simulink model "Example3_Calibrating_The_AR_Drone_Model"  (R2016a)
settings: configuration reference "AR_Drone_ConfigSet" (kept outside this file)
libraries: simulink x1, AR_Drone_2_Library x1, ARdrone_video_lib x1
settings Model: SimulationMode=external  Creator=sannem  LastModifiedBy=sannem
settings ConfigSetRef: SourceLocation=Base Workspace

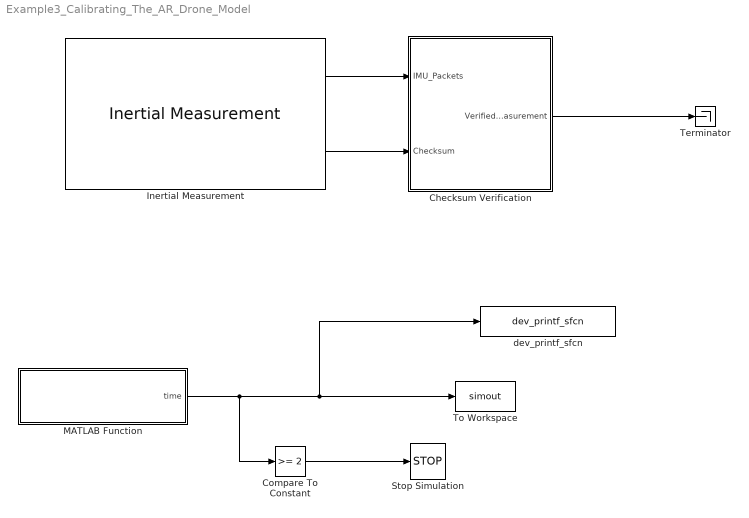
== system Example3_Calibrating_The_AR_Drone_Model ==
  Checksum Verification : Subsystem
  Compare To Constant : simulink/Logic and Bit Operations/Compare To Constant  relop=>=  const=2  OutDataTypeStr=boolean
  Inertial Measurement : AR_Drone_2_Library/Inertial Measurement  Ts=1/400
  MATLAB Function : MATLAB Function  TreatAsAtomicUnit=on
  Stop Simulation : Stop
  Terminator : Terminator
  To Workspace : ToWorkspace  VariableName=simout  SaveFormat=Structure With Time  SampleTime=-1
  dev_printf_sfcn : ARdrone_video_lib/dev_printf_sfcn  SFunctionSpec=ARpintf_Update(double u1)  SampleTime=-1  ShowSpec=on
  wires:
  Inertial Measurement/1 -> Checksum Verification/1(IMU_Packets)
  Inertial Measurement/2 -> Checksum Verification/2(Checksum)
  Checksum Verification/1(Verified_Raw_Measurement) -> Terminator/1
  MATLAB Function/1(time) -> Compare To Constant/1, To Workspace/1, dev_printf_sfcn/1
  Compare To Constant/1 -> Stop Simulation/1

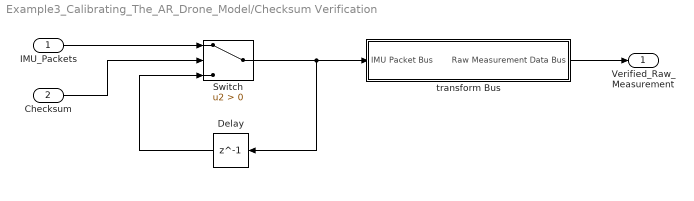
== system Example3_Calibrating_The_AR_Drone_Model/Checksum Verification ==
  IMU_Packets : Inport
  Checksum : Inport  Port=2
  Delay : Delay  DelayLength=1
  Switch : Switch  Criteria=u2 > Threshold
  transform Bus : Subsystem
  Verified_Raw_Measurement : Outport
  wires:
  IMU_Packets/1 -> Switch/1
  transform Bus/1(Raw Measurement Data Bus) -> Verified_Raw_Measurement/1
  Checksum/1 -> Switch/2
  Delay/1 -> Switch/3
  Switch/1 -> Delay/1, transform Bus/1(IMU Packet Bus)

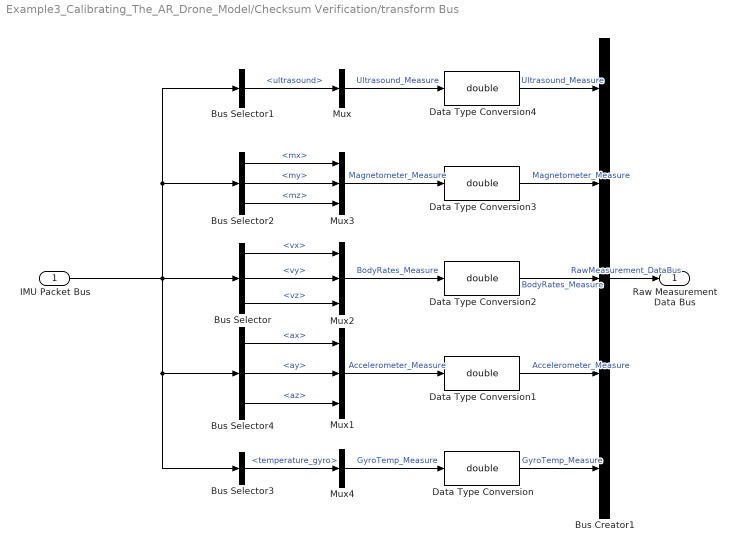
== system Example3_Calibrating_The_AR_Drone_Model/Checksum Verification/transform Bus ==
  IMU Packet Bus : Inport  OutDataTypeStr=Bus: IMU_Packets
  Bus Creator1 : BusCreator  Inputs='Ultrasound_Measure','Magnetometer_Measure','BodyRates_Measure','Accelerometer_Measure','GyroTemp_Measure'
  Bus Selector : BusSelector  OutputSignals=vx,vy,vz
  Bus Selector1 : BusSelector  OutputSignals=ultrasound
  Bus Selector2 : BusSelector  OutputSignals=mx,my,mz
  Bus Selector3 : BusSelector  OutputSignals=temperature_gyro
  Bus Selector4 : BusSelector  OutputSignals=ax,ay,az
  Data Type Conversion{,1..4} (5 alike) : DataTypeConversion  OutDataTypeStr=double
  Mux : Mux  Inputs=1
  Mux1 : Mux  Inputs=3
  Mux2 : Mux  Inputs=3
  Mux3 : Mux  Inputs=3
  Mux4 : Mux  Inputs=1
  Raw Measurement Data Bus : Outport
  wires:
  Bus Creator1/1 -> Raw Measurement Data Bus/1  "RawMeasurement_DataBus"
  Data Type Conversion3/1 -> Bus Creator1/2  "Magnetometer_Measure"
  Data Type Conversion1/1 -> Bus Creator1/4  "Accelerometer_Measure"
  Data Type Conversion2/1 -> Bus Creator1/3  "BodyRates_Measure"
  Bus Selector/3 -> Mux2/3  "<vz>"
  Bus Selector/2 -> Mux2/2  "<vy>"
  Bus Selector/1 -> Mux2/1  "<vx>"
  Bus Selector2/3 -> Mux3/3  "<mz>"
  Bus Selector2/2 -> Mux3/2  "<my>"
  Bus Selector2/1 -> Mux3/1  "<mx>"
  Bus Selector4/3 -> Mux1/3  "<az>"
  Bus Selector4/2 -> Mux1/2  "<ay>"
  Bus Selector4/1 -> Mux1/1  "<ax>"
  IMU Packet Bus/1 -> Bus Selector3/1, Bus Selector4/1, Bus Selector/1, Bus Selector1/1, Bus Selector2/1
  Bus Selector1/1 -> Mux/1  "<ultrasound>"
  Data Type Conversion4/1 -> Bus Creator1/1  "Ultrasound_Measure"
  Bus Selector3/1 -> Mux4/1  "<temperature_gyro>"
  Data Type Conversion/1 -> Bus Creator1/5  "GyroTemp_Measure"
  Mux4/1 -> Data Type Conversion/1  "GyroTemp_Measure"
  Mux1/1 -> Data Type Conversion1/1  "Accelerometer_Measure"
  Mux2/1 -> Data Type Conversion2/1  "BodyRates_Measure"
  Mux3/1 -> Data Type Conversion3/1  "Magnetometer_Measure"
  Mux/1 -> Data Type Conversion4/1  "Ultrasound_Measure"

== matlab function Example3_Calibrating_The_AR_Drone_Model/MATLAB Function ==
  data: time output
function time = shittyTempClock()
%#codegen

persistent runTime
if isempty(runTime)
   runTime = 0; 
else
   runTime = runTime + 1/400; 
end

time = runTime;
